simulink model "gm_uz_d_inverter_adapter"  (R2024b)
settings: Solver=FixedStepDiscrete  StartTime=0.0  StopTime=300e-5  RelTol=1e-3
undefined symbols (not defined in the file or in its folder): t_clk, t_clk_sig
libraries: hdlsllib x16, simulink x12
settings Model: Creator=Michael Hoerner  LastModifiedBy=hufnagelde
settings SolverCC: AlgebraicLoopSolver=TrustRegion
settings DataIOCC: LimitDataPoints=on  SaveOutput=off  SaveTime=off
settings OptimizationCC: BlockReduction=off  ConditionallyExecuteInputs=off  DefaultParameterBehavior=Inlined  LifeSpan=inf
settings DebuggingCC: AlgebraicLoopMsg=error  InheritedTsInSrcMsg=none  SingleTaskRateTransMsg=warning  UnconnectedInputMsg=warning  UnconnectedOutputMsg=warning  UnconnectedLineMsg=warning  AllowSymbolicDim=off  StrictBusMsg=ErrorOnBusTreatedAsVector  SFUnexpectedBacktrackingDiag=warning  SFNoUnconditionalDefaultTransitionDiag=warning  SFExecutionAtInitializationDiag=none  ArithmeticOperatorsInVariantConditions=warning
settings HardwareCC: ProdBitPerPointer=32  ProdBitPerSizeT=32  ProdBitPerPtrDiffT=32  ProdLargestAtomicFloat=None  ProdIntDivRoundTo=Undefined  ProdEndianess=Unspecified  ProdWordSize=32  ProdHWDeviceType=ASIC/FPGA->ASIC/FPGA  ProdEqTarget=off
settings ModelReferenceCC: EnableRefExpFcnMdlSchedulingChecks=on
settings SFSimCC: SimUseLocalCustomCode=off  CustomCodeUndefinedFunction=UseInterfaceOnly
settings RTWCC: RTWUseLocalCustomCode=off  GPUComputeCapability=3.5  DLArmComputeVersion=19.05
settings CodeAppCC: StateflowObjectComments=on
settings GRTTargetCC: TargetLangStandard=C89/C90 (ANSI)
settings ConfigComp: CovScope=ReferencedModels  CovMetricSettings=dw  CovSaveCumulativeToWorkspaceVar=on  CovSaveSingleToWorkspaceVar=on  CovExternalEMLEnable=off  CovSFcnEnable=off

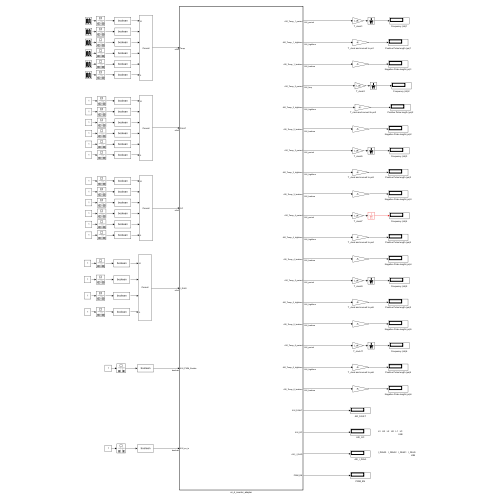
[thumbnail: Simulink's stored preview of the top-level diagram]
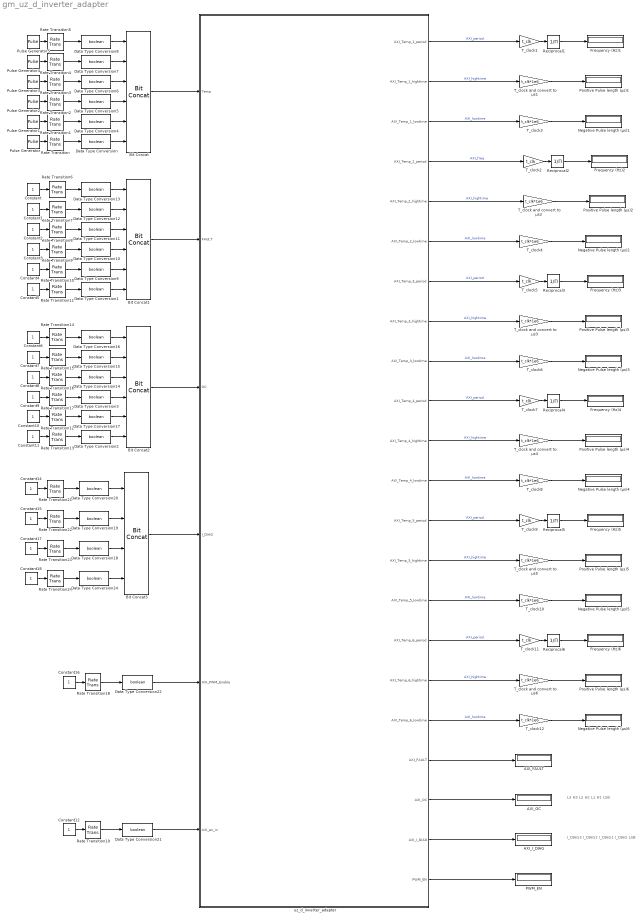
== system gm_uz_d_inverter_adapter ==
  note: I_DIAG3   I_DIAG2   I_DIAG1   I_DIAG
      |                                                        LSB
  note: L3   H3   L2   H2   L1   H1
      |                                   LSB
  AXI_FAULT : Display
      settings: Format=binary (Stored Integer)
  AXI_I_DIAG : Display
      settings: Format=binary (Stored Integer)
  AXI_OC : Display
      settings: Format=binary (Stored Integer)
  Bit Concat : hdlsllib/Logic and Bit Operations/Bit Concat  numInputs=6
  Bit Concat1 : hdlsllib/Logic and Bit Operations/Bit Concat  numInputs=6
  Bit Concat2 : hdlsllib/Logic and Bit Operations/Bit Concat  numInputs=6
  Bit Concat3 : hdlsllib/Logic and Bit Operations/Bit Concat  numInputs=4
  Constant{,1..12,14..18} (18 alike) : Constant
  Data Type Conversion{,1..22,24} (24 alike) : DataTypeConversion  OutDataTypeStr=boolean  SaturateOnIntegerOverflow=off  RndMeth=Floor
  Frequency (Hz){1..6} (6 alike) : Display
  Negative Pulse length (µs){1..6} (6 alike) : Display
  PWM_EN : Display
      settings: Format=decimal (Stored Integer)
  Positive Pulse length (µs){1..6} (6 alike) : Display
  Pulse Generator : DiscretePulseGenerator  PulseType=Time based  Period=t_clk_sig  PulseWidth=10
  Pulse Generator1 : DiscretePulseGenerator  PulseType=Time based  Period=t_clk_sig  PulseWidth=20
  Pulse Generator2 : DiscretePulseGenerator  PulseType=Time based  Period=t_clk_sig  PulseWidth=30
  Pulse Generator3 : DiscretePulseGenerator  PulseType=Time based  Period=t_clk_sig  PulseWidth=40
  Pulse Generator4 : DiscretePulseGenerator  PulseType=Time based  Period=t_clk_sig  PulseWidth=50
  Pulse Generator5 : DiscretePulseGenerator  PulseType=Time based  Period=t_clk_sig  PulseWidth=60
  Rate Transition{,1..5} (6 alike) : RateTransition  Deterministic=off  OutPortSampleTime=t_clk
  Rate Transition{6..19,21..24} (18 alike) : RateTransition  OutPortSampleTime=t_clk
  Reciprocal{1..6} (6 alike) : Product  Inputs=/
  T_clock and convert to µs{1..6} (6 alike) : Gain  Gain=t_clk*1e6
  T_clock{1..2,5,7,9,11} (6 alike) : Gain  Gain=t_clk
  T_clock{3..4,6,8,10,12} (6 alike) : Gain  Gain=t_clk*1e6
  uz_d_inverter_adapter : Subsystem  TreatAsAtomicUnit=on
  wires:
  Data Type Conversion21/1 -> uz_d_inverter_adapter/6(AXI_en_in)
  Rate Transition19/1 -> Data Type Conversion21/1
  Constant12/1 -> Rate Transition19/1
  uz_d_inverter_adapter/22(PWM_EN) -> PWM_EN/1
  uz_d_inverter_adapter/21(AXI_I_DIAG) -> AXI_I_DIAG/1
  uz_d_inverter_adapter/20(AXI_OC) -> AXI_OC/1
  Bit Concat3/1 -> uz_d_inverter_adapter/4(I_DIAG)
  Data Type Conversion24/1 -> Bit Concat3/4
  Data Type Conversion18/1 -> Bit Concat3/3
  Data Type Conversion19/1 -> Bit Concat3/2
  Data Type Conversion20/1 -> Bit Concat3/1
  Rate Transition23/1 -> Data Type Conversion18/1
  Rate Transition21/1 -> Data Type Conversion20/1
  Rate Transition24/1 -> Data Type Conversion24/1
  Constant17/1 -> Rate Transition23/1
  Constant14/1 -> Rate Transition21/1
  Rate Transition22/1 -> Data Type Conversion19/1
  Constant15/1 -> Rate Transition22/1
  Constant18/1 -> Rate Transition24/1
  Bit Concat2/1 -> uz_d_inverter_adapter/3(OC)
  Data Type Conversion2/1 -> Bit Concat2/6
  Constant7/1 -> Rate Transition15/1
  Rate Transition15/1 -> Data Type Conversion15/1
  Constant9/1 -> Rate Transition17/1
  Data Type Conversion17/1 -> Bit Concat2/5
  Constant10/1 -> Rate Transition12/1
  Constant11/1 -> Rate Transition13/1
  Constant8/1 -> Rate Transition16/1
  Constant6/1 -> Rate Transition14/1
  Rate Transition12/1 -> Data Type Conversion17/1
  Data Type Conversion15/1 -> Bit Concat2/2
  Data Type Conversion14/1 -> Bit Concat2/3
  Data Type Conversion3/1 -> Bit Concat2/4
  Rate Transition13/1 -> Data Type Conversion2/1
  Rate Transition14/1 -> Data Type Conversion16/1
  Rate Transition17/1 -> Data Type Conversion3/1
  Rate Transition16/1 -> Data Type Conversion14/1
  Data Type Conversion16/1 -> Bit Concat2/1
  Data Type Conversion22/1 -> uz_d_inverter_adapter/5(AXI_PWM_Enable)
  Rate Transition11/1 -> Data Type Conversion1/1
  Rate Transition10/1 -> Data Type Conversion9/1
  Rate Transition9/1 -> Data Type Conversion10/1
  Rate Transition8/1 -> Data Type Conversion11/1
  Rate Transition7/1 -> Data Type Conversion12/1
  Rate Transition6/1 -> Data Type Conversion13/1
  Bit Concat1/1 -> uz_d_inverter_adapter/2(FAULT)
  Data Type Conversion1/1 -> Bit Concat1/6
  Data Type Conversion13/1 -> Bit Concat1/1
  Data Type Conversion12/1 -> Bit Concat1/2
  Data Type Conversion9/1 -> Bit Concat1/5
  Data Type Conversion10/1 -> Bit Concat1/4
  Data Type Conversion11/1 -> Bit Concat1/3
  Data Type Conversion4/1 -> Bit Concat/5
  Data Type Conversion/1 -> Bit Concat/6
  Rate Transition5/1 -> Data Type Conversion8/1
  Rate Transition4/1 -> Data Type Conversion7/1
  Rate Transition3/1 -> Data Type Conversion6/1
  Rate Transition2/1 -> Data Type Conversion5/1
  Rate Transition1/1 -> Data Type Conversion4/1
  Bit Concat/1 -> uz_d_inverter_adapter/1(Temp)
  Rate Transition18/1 -> Data Type Conversion22/1
  Constant16/1 -> Rate Transition18/1
  Data Type Conversion8/1 -> Bit Concat/1
  Data Type Conversion7/1 -> Bit Concat/2
  Data Type Conversion6/1 -> Bit Concat/3
  Data Type Conversion5/1 -> Bit Concat/4
  uz_d_inverter_adapter/19(AXI_FAULT) -> AXI_FAULT/1
  uz_d_inverter_adapter/16(AXI_Temp_6_period) -> T_clock11/1  "AXI_period"
  T_clock and convert to µs6/1 -> Positive Pulse length (µs)6/1
  uz_d_inverter_adapter/17(AXI_Temp_6_hightime) -> T_clock and convert to µs6/1  "AXI_hightime"
  T_clock12/1 -> Negative Pulse length (µs)6/1
  Reciprocal6/1 -> Frequency (Hz)6/1
  T_clock11/1 -> Reciprocal6/1
  uz_d_inverter_adapter/18(AXI_Temp_6_lowtime) -> T_clock12/1  "AXI_lowtime"
  uz_d_inverter_adapter/13(AXI_Temp_5_period) -> T_clock9/1  "AXI_period"
  T_clock and convert to µs5/1 -> Positive Pulse length (µs)5/1
  uz_d_inverter_adapter/14(AXI_Temp_5_hightime) -> T_clock and convert to µs5/1  "AXI_hightime"
  T_clock10/1 -> Negative Pulse length (µs)5/1
  Reciprocal5/1 -> Frequency (Hz)5/1
  T_clock9/1 -> Reciprocal5/1
  uz_d_inverter_adapter/15(AXI_Temp_5_lowtime) -> T_clock10/1  "AXI_lowtime"
  uz_d_inverter_adapter/10(AXI_Temp_4_period) -> T_clock7/1  "AXI_period"
  T_clock and convert to µs4/1 -> Positive Pulse length (µs)4/1
  uz_d_inverter_adapter/11(AXI_Temp_4_hightime) -> T_clock and convert to µs4/1  "AXI_hightime"
  T_clock8/1 -> Negative Pulse length (µs)4/1
  Reciprocal4/1 -> Frequency (Hz)4/1
  T_clock7/1 -> Reciprocal4/1
  uz_d_inverter_adapter/12(AXI_Temp_4_lowtime) -> T_clock8/1  "AXI_lowtime"
  uz_d_inverter_adapter/7(AXI_Temp_3_period) -> T_clock5/1  "AXI_period"
  T_clock and convert to µs3/1 -> Positive Pulse length (µs)3/1
  uz_d_inverter_adapter/8(AXI_Temp_3_hightime) -> T_clock and convert to µs3/1  "AXI_hightime"
  T_clock6/1 -> Negative Pulse length (µs)3/1
  Reciprocal3/1 -> Frequency (Hz)3/1
  T_clock5/1 -> Reciprocal3/1
  uz_d_inverter_adapter/9(AXI_Temp_3_lowtime) -> T_clock6/1  "AXI_lowtime"
  uz_d_inverter_adapter/4(AXI_Temp_2_period) -> T_clock2/1  "AXI_freq"
  T_clock and convert to µs2/1 -> Positive Pulse length (µs)2/1
  uz_d_inverter_adapter/5(AXI_Temp_2_hightime) -> T_clock and convert to µs2/1  "AXI_hightime"
  T_clock4/1 -> Negative Pulse length (µs)2/1
  Reciprocal2/1 -> Frequency (Hz)2/1
  T_clock2/1 -> Reciprocal2/1
  uz_d_inverter_adapter/6(AXI_Temp_2_lowtime) -> T_clock4/1  "AXI_lowtime"
  uz_d_inverter_adapter/1(AXI_Temp_1_period) -> T_clock1/1  "AXI_period"
  T_clock1/1 -> Reciprocal1/1
  uz_d_inverter_adapter/2(AXI_Temp_1_hightime) -> T_clock and convert to µs1/1  "AXI_hightime"
  uz_d_inverter_adapter/3(AXI_Temp_1_lowtime) -> T_clock3/1  "AXI_lowtime"
  Reciprocal1/1 -> Frequency (Hz)1/1
  T_clock3/1 -> Negative Pulse length (µs)1/1
  T_clock and convert to µs1/1 -> Positive Pulse length (µs)1/1
  Constant5/1 -> Rate Transition11/1
  Constant4/1 -> Rate Transition10/1
  Constant3/1 -> Rate Transition9/1
  Constant2/1 -> Rate Transition8/1
  Constant1/1 -> Rate Transition7/1
  Constant/1 -> Rate Transition6/1
  Rate Transition/1 -> Data Type Conversion/1
  Pulse Generator5/1 -> Rate Transition5/1
  Pulse Generator4/1 -> Rate Transition4/1
  Pulse Generator3/1 -> Rate Transition3/1
  Pulse Generator2/1 -> Rate Transition2/1
  Pulse Generator1/1 -> Rate Transition1/1
  Pulse Generator/1 -> Rate Transition/1

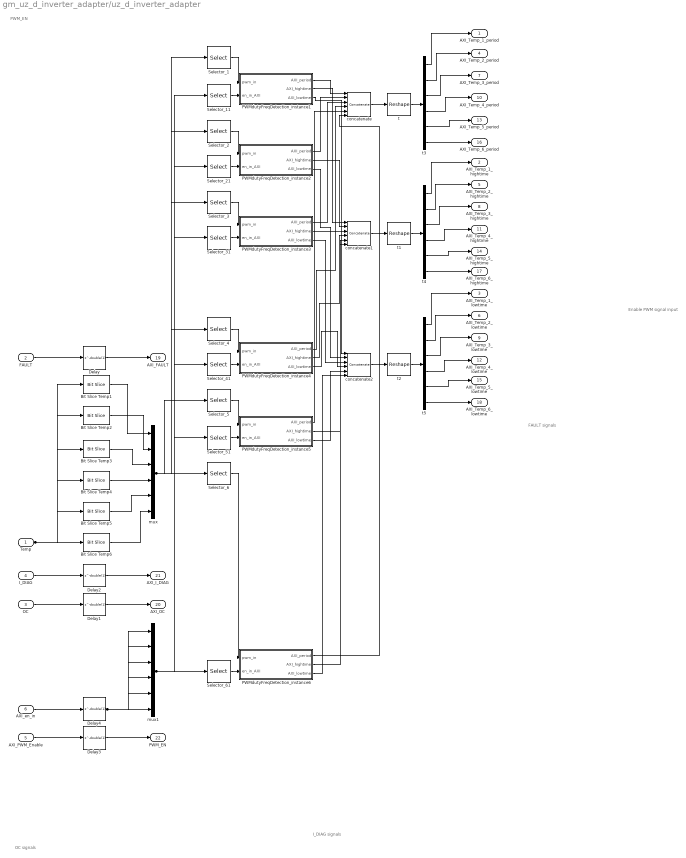
== system gm_uz_d_inverter_adapter/uz_d_inverter_adapter ==
  note: PWM_EN
  note: I_DIAG signals
  note: FAULT signals
  note: OC signals
  note: Enable PWM signal input
  Temp : Inport  OutDataTypeStr=fixdt(0, 6, 0)  PortDimensions=1  SampleTime=1e-08
  FAULT : Inport  Port=2  OutDataTypeStr=fixdt(0, 6, 0)  PortDimensions=1  SampleTime=1e-08
  OC : Inport  Port=3  OutDataTypeStr=fixdt(0, 6, 0)  PortDimensions=1  SampleTime=1e-08
  I_DIAG : Inport  Port=4  OutDataTypeStr=fixdt(0, 4, 0)  PortDimensions=1  SampleTime=1e-08
  AXI_PWM_Enable : Inport  Port=5  OutDataTypeStr=boolean  PortDimensions=1  SampleTime=1e-08
  AXI_en_in : Inport  Port=6  OutDataTypeStr=boolean  PortDimensions=1  SampleTime=1e-08
  Bit Slice Temp1 : hdlsllib/Logic and Bit Operations/Bit Slice  lidx=double(0)  ridx=double(0)
  Bit Slice Temp2 : hdlsllib/Logic and Bit Operations/Bit Slice  lidx=double(1)  ridx=double(1)
  Bit Slice Temp3 : hdlsllib/Logic and Bit Operations/Bit Slice  lidx=double(2)  ridx=double(2)
  Bit Slice Temp4 : hdlsllib/Logic and Bit Operations/Bit Slice  lidx=double(3)  ridx=double(3)
  Bit Slice Temp5 : hdlsllib/Logic and Bit Operations/Bit Slice  lidx=double(4)  ridx=double(4)
  Bit Slice Temp6 : hdlsllib/Logic and Bit Operations/Bit Slice  lidx=double(5)  ridx=double(5)
  Delay{,1..4} (5 alike) : Delay  DelayLength=double(1)  InitialCondition=0  SampleTime=1e-08
  PWMdutyFreqDetection_instance1 : Subsystem
  PWMdutyFreqDetection_instance2 : Subsystem
  PWMdutyFreqDetection_instance3 : Subsystem
  PWMdutyFreqDetection_instance4 : Subsystem
  PWMdutyFreqDetection_instance5 : Subsystem
  PWMdutyFreqDetection_instance6 : Subsystem
  Selector_1 : Selector  InputPortWidth=6  IndexOptions=Index vector (dialog)  Indices=double(1)  OutputSizes=1
  Selector_11 : Selector  InputPortWidth=6  IndexOptions=Index vector (dialog)  Indices=double(1)  OutputSizes=1
  Selector_2 : Selector  InputPortWidth=6  IndexOptions=Index vector (dialog)  Indices=double(2)  OutputSizes=1
  Selector_21 : Selector  InputPortWidth=6  IndexOptions=Index vector (dialog)  Indices=double(2)  OutputSizes=1
  Selector_3 : Selector  InputPortWidth=6  IndexOptions=Index vector (dialog)  Indices=double(3)  OutputSizes=1
  Selector_31 : Selector  InputPortWidth=6  IndexOptions=Index vector (dialog)  Indices=double(3)  OutputSizes=1
  Selector_4 : Selector  InputPortWidth=6  IndexOptions=Index vector (dialog)  Indices=double(4)  OutputSizes=1
  Selector_41 : Selector  InputPortWidth=6  IndexOptions=Index vector (dialog)  Indices=double(4)  OutputSizes=1
  Selector_5 : Selector  InputPortWidth=6  IndexOptions=Index vector (dialog)  Indices=double(5)  OutputSizes=1
  Selector_51 : Selector  InputPortWidth=6  IndexOptions=Index vector (dialog)  Indices=double(5)  OutputSizes=1
  Selector_6 : Selector  InputPortWidth=6  IndexOptions=Index vector (dialog)  Indices=double(6)  OutputSizes=1
  Selector_61 : Selector  InputPortWidth=6  IndexOptions=Index vector (dialog)  Indices=double(6)  OutputSizes=1
  concatenate : Concatenate  NumInputs=6
  concatenate1 : Concatenate  NumInputs=6
  concatenate2 : Concatenate  NumInputs=6
  mux : Mux  Inputs=6
  mux1 : Mux  Inputs=6
  t : Reshape
  t1 : Reshape
  t2 : Reshape
  t3 : Demux  Outputs=6
  t4 : Demux  Outputs=6
  t5 : Demux  Outputs=6
  AXI_Temp_1_period : Outport  PortDimensions=1  SampleTime=1e-08  VectorParamsAs1DForOutWhenUnconnected=off
  AXI_Temp_1_hightime : Outport  Port=2  PortDimensions=1  SampleTime=1e-08  VectorParamsAs1DForOutWhenUnconnected=off
  AXI_Temp_1_lowtime : Outport  Port=3  PortDimensions=1  SampleTime=1e-08  VectorParamsAs1DForOutWhenUnconnected=off
  AXI_Temp_2_period : Outport  Port=4  PortDimensions=1  SampleTime=1e-08  VectorParamsAs1DForOutWhenUnconnected=off
  AXI_Temp_2_hightime : Outport  Port=5  PortDimensions=1  SampleTime=1e-08  VectorParamsAs1DForOutWhenUnconnected=off
  AXI_Temp_2_lowtime : Outport  Port=6  PortDimensions=1  SampleTime=1e-08  VectorParamsAs1DForOutWhenUnconnected=off
  AXI_Temp_3_period : Outport  Port=7  PortDimensions=1  SampleTime=1e-08  VectorParamsAs1DForOutWhenUnconnected=off
  AXI_Temp_3_hightime : Outport  Port=8  PortDimensions=1  SampleTime=1e-08  VectorParamsAs1DForOutWhenUnconnected=off
  AXI_Temp_3_lowtime : Outport  Port=9  PortDimensions=1  SampleTime=1e-08  VectorParamsAs1DForOutWhenUnconnected=off
  AXI_Temp_4_period : Outport  Port=10  PortDimensions=1  SampleTime=1e-08  VectorParamsAs1DForOutWhenUnconnected=off
  AXI_Temp_4_hightime : Outport  Port=11  PortDimensions=1  SampleTime=1e-08  VectorParamsAs1DForOutWhenUnconnected=off
  AXI_Temp_4_lowtime : Outport  Port=12  PortDimensions=1  SampleTime=1e-08  VectorParamsAs1DForOutWhenUnconnected=off
  AXI_Temp_5_period : Outport  Port=13  PortDimensions=1  SampleTime=1e-08  VectorParamsAs1DForOutWhenUnconnected=off
  AXI_Temp_5_hightime : Outport  Port=14  PortDimensions=1  SampleTime=1e-08  VectorParamsAs1DForOutWhenUnconnected=off
  AXI_Temp_5_lowtime : Outport  Port=15  PortDimensions=1  SampleTime=1e-08  VectorParamsAs1DForOutWhenUnconnected=off
  AXI_Temp_6_period : Outport  Port=16  PortDimensions=1  SampleTime=1e-08  VectorParamsAs1DForOutWhenUnconnected=off
  AXI_Temp_6_hightime : Outport  Port=17  PortDimensions=1  SampleTime=1e-08  VectorParamsAs1DForOutWhenUnconnected=off
  AXI_Temp_6_lowtime : Outport  Port=18  PortDimensions=1  SampleTime=1e-08  VectorParamsAs1DForOutWhenUnconnected=off
  AXI_FAULT : Outport  Port=19  PortDimensions=1  SampleTime=1e-08  VectorParamsAs1DForOutWhenUnconnected=off
  AXI_OC : Outport  Port=20  PortDimensions=1  SampleTime=1e-08  VectorParamsAs1DForOutWhenUnconnected=off
  AXI_I_DIAG : Outport  Port=21  PortDimensions=1  SampleTime=1e-08  VectorParamsAs1DForOutWhenUnconnected=off
  PWM_EN : Outport  Port=22  PortDimensions=1  SampleTime=1e-08  VectorParamsAs1DForOutWhenUnconnected=off
  wires:
  PWMdutyFreqDetection_instance4/3(AXI_lowtime) -> concatenate2/4
  Delay/1 -> AXI_FAULT/1
  t3/2 -> AXI_Temp_2_period/1
  PWMdutyFreqDetection_instance3/1(AXI_period) -> concatenate/3
  t3/1 -> AXI_Temp_1_period/1
  FAULT/1 -> Delay/1
  PWMdutyFreqDetection_instance4/1(AXI_period) -> concatenate/4
  Selector_51/1 -> PWMdutyFreqDetection_instance5/2(en_in_AXI)
  Temp/1 -> Bit Slice Temp6/1, Bit Slice Temp5/1, Bit Slice Temp4/1, Bit Slice Temp3/1, Bit Slice Temp1/1, Bit Slice Temp2/1
  AXI_en_in/1 -> Delay4/1
  I_DIAG/1 -> Delay2/1
  OC/1 -> Delay1/1
  AXI_PWM_Enable/1 -> Delay3/1
  Selector_21/1 -> PWMdutyFreqDetection_instance2/2(en_in_AXI)
  Bit Slice Temp1/1 -> mux/1
  Bit Slice Temp2/1 -> mux/2
  Bit Slice Temp3/1 -> mux/3
  Selector_11/1 -> PWMdutyFreqDetection_instance1/2(en_in_AXI)
  Bit Slice Temp4/1 -> mux/4
  PWMdutyFreqDetection_instance2/1(AXI_period) -> concatenate/2
  Bit Slice Temp5/1 -> mux/5
  PWMdutyFreqDetection_instance6/2(AXI_hightime) -> concatenate1/6
  Bit Slice Temp6/1 -> mux/6
  Selector_4/1 -> PWMdutyFreqDetection_instance4/1(pwm_in)
  Delay2/1 -> AXI_I_DIAG/1
  t3/4 -> AXI_Temp_4_period/1
  Delay1/1 -> AXI_OC/1
  t3/3 -> AXI_Temp_3_period/1
  Selector_6/1 -> PWMdutyFreqDetection_instance6/1(pwm_in)
  Delay4/1 -> mux1/3, mux1/2, mux1/1, mux1/4, mux1/5, mux1/6
  Delay3/1 -> PWM_EN/1
  mux/1 -> Selector_3/1, Selector_6/1, Selector_2/1, Selector_1/1, Selector_4/1, Selector_5/1
  mux1/1 -> Selector_61/1, Selector_41/1, Selector_51/1, Selector_21/1, Selector_11/1, Selector_31/1
  Selector_1/1 -> PWMdutyFreqDetection_instance1/1(pwm_in)
  PWMdutyFreqDetection_instance5/2(AXI_hightime) -> concatenate1/5
  Selector_2/1 -> PWMdutyFreqDetection_instance2/1(pwm_in)
  Selector_3/1 -> PWMdutyFreqDetection_instance3/1(pwm_in)
  Selector_31/1 -> PWMdutyFreqDetection_instance3/2(en_in_AXI)
  Selector_41/1 -> PWMdutyFreqDetection_instance4/2(en_in_AXI)
  Selector_5/1 -> PWMdutyFreqDetection_instance5/1(pwm_in)
  t3/6 -> AXI_Temp_6_period/1
  t3/5 -> AXI_Temp_5_period/1
  Selector_61/1 -> PWMdutyFreqDetection_instance6/2(en_in_AXI)
  PWMdutyFreqDetection_instance1/1(AXI_period) -> concatenate/1
  PWMdutyFreqDetection_instance1/2(AXI_hightime) -> concatenate1/1
  PWMdutyFreqDetection_instance5/3(AXI_lowtime) -> concatenate2/5
  PWMdutyFreqDetection_instance1/3(AXI_lowtime) -> concatenate2/1
  PWMdutyFreqDetection_instance6/1(AXI_period) -> concatenate/6
  PWMdutyFreqDetection_instance2/2(AXI_hightime) -> concatenate1/2
  PWMdutyFreqDetection_instance6/3(AXI_lowtime) -> concatenate2/6
  PWMdutyFreqDetection_instance2/3(AXI_lowtime) -> concatenate2/2
  PWMdutyFreqDetection_instance3/2(AXI_hightime) -> concatenate1/3
  PWMdutyFreqDetection_instance3/3(AXI_lowtime) -> concatenate2/3
  PWMdutyFreqDetection_instance4/2(AXI_hightime) -> concatenate1/4
  PWMdutyFreqDetection_instance5/1(AXI_period) -> concatenate/5
  concatenate/1 -> t/1
  concatenate1/1 -> t1/1
  concatenate2/1 -> t2/1
  t/1 -> t3/1
  t1/1 -> t4/1
  t2/1 -> t5/1
  t4/2 -> AXI_Temp_2_hightime/1
  t4/1 -> AXI_Temp_1_hightime/1
  t4/3 -> AXI_Temp_3_hightime/1
  t4/4 -> AXI_Temp_4_hightime/1
  t4/5 -> AXI_Temp_5_hightime/1
  t4/6 -> AXI_Temp_6_hightime/1
  t5/1 -> AXI_Temp_1_lowtime/1
  t5/2 -> AXI_Temp_2_lowtime/1
  t5/3 -> AXI_Temp_3_lowtime/1
  t5/4 -> AXI_Temp_4_lowtime/1
  t5/5 -> AXI_Temp_5_lowtime/1
  t5/6 -> AXI_Temp_6_lowtime/1

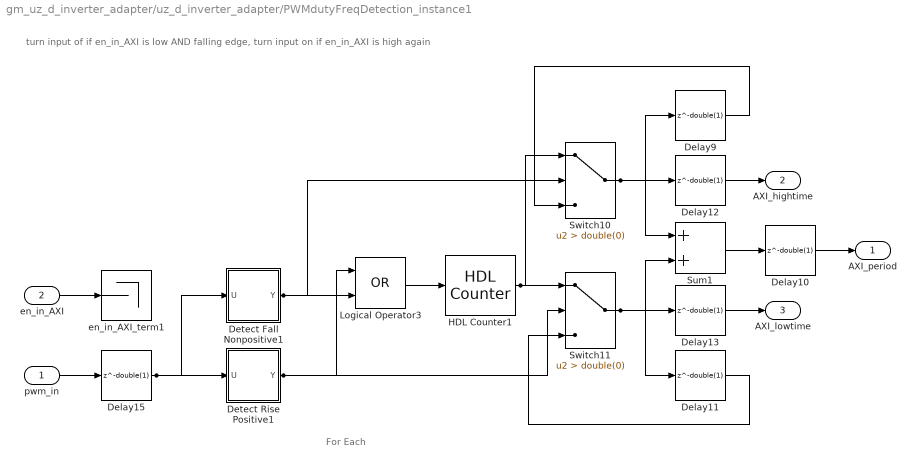
== system gm_uz_d_inverter_adapter/uz_d_inverter_adapter/PWMdutyFreqDetection_instance1 ==
  note: For Each
  note: turn input of if en_in_AXI is low AND falling edge, turn input on if en_in_AXI is high again
  pwm_in : Inport  OutDataTypeStr=fixdt(0, 1, 0)  PortDimensions=1  SampleTime=1e-08
  en_in_AXI : Inport  Port=2  OutDataTypeStr=boolean  PortDimensions=1  SampleTime=1e-08
  Delay{9..13,15} (6 alike) : Delay  DelayLength=double(1)  InitialCondition=0  SampleTime=1e-08
  Detect Fall Nonpositive1 : Subsystem  mask(Detect Fall Nonpositive){vinit=double(0), InputProcessing=Elements as channels (sample based), OutDataTypeStr=boolean}
      mask prompts: vinit "Simulink:masks:InitialCondition_MP"; InputProcessing "Simulink:masks:InputProcessing_MP"; OutDataTypeStr "Simulink:masks:OutputDataType_MP"
      mask help: Simulink:masks:DetectFallNonpositive_MD
      mask init:
      | InputProcessing = 'Elements as channels (sample based)';
      | OutDataTypeStr = 'boolean';
      | vinit = double(0);
      mask TypeOptions InputProcessing: Simulink:masks:ColumnsAsChannelsFrameBased | Simulink:masks:ElementsAsChannelsSampleBased
      mask TypeOptions OutDataTypeStr: Simulink:masks:uint8 | Simulink:masks:boolean
      mask Display: fprintf('U <= 0\n&  NOT\nU/z <= 0')
  Detect Rise Positive1 : Subsystem  mask(Detect Rise Positive){vinit=double(0), InputProcessing=Elements as channels (sample based), OutDataTypeStr=boolean}
      mask prompts: vinit "Simulink:masks:InitialCondition_MP"; InputProcessing "Simulink:masks:InputProcessing_MP"; OutDataTypeStr "Simulink:masks:OutputDataType_MP"
      mask help: Simulink:masks:DetectRisePositive_MD
      mask init:
      | InputProcessing = 'Elements as channels (sample based)';
      | OutDataTypeStr = 'boolean';
      | vinit = double(0);
      mask TypeOptions InputProcessing: Simulink:masks:ColumnsAsChannelsFrameBased | Simulink:masks:ElementsAsChannelsSampleBased
      mask TypeOptions OutDataTypeStr: Simulink:masks:uint8 | Simulink:masks:boolean
      mask Display: fprintf('U > 0\n&  NOT\nU/z > 0')
  HDL Counter1 : hdlsllib/Sources/HDL Counter  CountType=Count limited  CountInit=1  CountStep=1  CountMax=2500000  CountFromType=Specify  CountFrom=1  CountResetPort=on  CountLoadPort=off  CountEnbPort=off  CountDirPort=off  CountHitOutputPort=off  CountDataType=Unsigned  CountWordLen=32  CountFracLen=0  CountSampTime=1
  Logical Operator3 : Logic  Operator=OR  AllPortsSameDT=off  OutDataTypeStr=boolean  SampleTime=1e-08
  Sum1 : Sum  OutDataTypeStr=uint32  AccumDataTypeStr=uint32  SampleTime=1e-08
  Switch10 : Switch  Criteria=u2 > Threshold  Threshold=double(0)  OutDataTypeStr=uint32  SampleTime=1e-08  SaturateOnIntegerOverflow=off  InputSameDT=off
  Switch11 : Switch  Criteria=u2 > Threshold  Threshold=double(0)  OutDataTypeStr=uint32  SampleTime=1e-08  SaturateOnIntegerOverflow=off  InputSameDT=off
  en_in_AXI_term1 : Terminator
  AXI_period : Outport  SampleTime=1e-08
  AXI_hightime : Outport  Port=2  SampleTime=1e-08
  AXI_lowtime : Outport  Port=3  SampleTime=1e-08
  wires:
  en_in_AXI/1 -> en_in_AXI_term1/1
  Detect Fall Nonpositive1/1(Y) -> Switch10/2, Logical Operator3/2
  pwm_in/1 -> Delay15/1
  Switch10/1 -> Sum1/1, Delay12/1, Delay9/1
  Delay12/1 -> AXI_hightime/1
  Logical Operator3/1 -> HDL Counter1/1
  Delay15/1 -> Detect Fall Nonpositive1/1(U), Detect Rise Positive1/1(U)
  Detect Rise Positive1/1(Y) -> Switch11/2, Logical Operator3/1
  HDL Counter1/1 -> Switch10/1, Switch11/1
  Delay13/1 -> AXI_lowtime/1
  Switch11/1 -> Sum1/2, Delay13/1, Delay11/1
  Delay9/1 -> Switch10/3
  Sum1/1 -> Delay10/1
  Delay11/1 -> Switch11/3
  Delay10/1 -> AXI_period/1

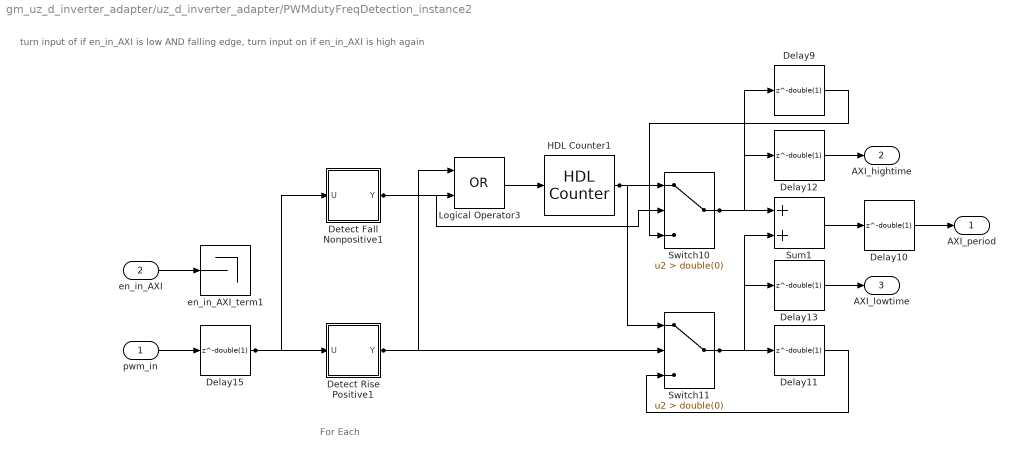
== system gm_uz_d_inverter_adapter/uz_d_inverter_adapter/PWMdutyFreqDetection_instance2 ==
  note: For Each
  note: turn input of if en_in_AXI is low AND falling edge, turn input on if en_in_AXI is high again
  pwm_in : Inport  OutDataTypeStr=fixdt(0, 1, 0)  PortDimensions=1  SampleTime=1e-08
  en_in_AXI : Inport  Port=2  OutDataTypeStr=boolean  PortDimensions=1  SampleTime=1e-08
  Delay{9..13,15} (6 alike) : Delay  DelayLength=double(1)  InitialCondition=0  SampleTime=1e-08
  Detect Fall Nonpositive1 : Subsystem  mask(Detect Fall Nonpositive){vinit=double(0), InputProcessing=Elements as channels (sample based), OutDataTypeStr=boolean}
      mask prompts: vinit "Simulink:masks:InitialCondition_MP"; InputProcessing "Simulink:masks:InputProcessing_MP"; OutDataTypeStr "Simulink:masks:OutputDataType_MP"
      mask help: Simulink:masks:DetectFallNonpositive_MD
      mask init:
      | InputProcessing = 'Elements as channels (sample based)';
      | OutDataTypeStr = 'boolean';
      | vinit = double(0);
      mask TypeOptions InputProcessing: Simulink:masks:ColumnsAsChannelsFrameBased | Simulink:masks:ElementsAsChannelsSampleBased
      mask TypeOptions OutDataTypeStr: Simulink:masks:uint8 | Simulink:masks:boolean
      mask Display: fprintf('U <= 0\n&  NOT\nU/z <= 0')
  Detect Rise Positive1 : Subsystem  mask(Detect Rise Positive){vinit=double(0), InputProcessing=Elements as channels (sample based), OutDataTypeStr=boolean}
      mask prompts: vinit "Simulink:masks:InitialCondition_MP"; InputProcessing "Simulink:masks:InputProcessing_MP"; OutDataTypeStr "Simulink:masks:OutputDataType_MP"
      mask help: Simulink:masks:DetectRisePositive_MD
      mask init:
      | InputProcessing = 'Elements as channels (sample based)';
      | OutDataTypeStr = 'boolean';
      | vinit = double(0);
      mask TypeOptions InputProcessing: Simulink:masks:ColumnsAsChannelsFrameBased | Simulink:masks:ElementsAsChannelsSampleBased
      mask TypeOptions OutDataTypeStr: Simulink:masks:uint8 | Simulink:masks:boolean
      mask Display: fprintf('U > 0\n&  NOT\nU/z > 0')
  HDL Counter1 : hdlsllib/Sources/HDL Counter  CountType=Count limited  CountInit=1  CountStep=1  CountMax=2500000  CountFromType=Specify  CountFrom=1  CountResetPort=on  CountLoadPort=off  CountEnbPort=off  CountDirPort=off  CountHitOutputPort=off  CountDataType=Unsigned  CountWordLen=32  CountFracLen=0  CountSampTime=1
  Logical Operator3 : Logic  Operator=OR  AllPortsSameDT=off  OutDataTypeStr=boolean  SampleTime=1e-08
  Sum1 : Sum  OutDataTypeStr=uint32  AccumDataTypeStr=uint32  SampleTime=1e-08
  Switch10 : Switch  Criteria=u2 > Threshold  Threshold=double(0)  OutDataTypeStr=uint32  SampleTime=1e-08  SaturateOnIntegerOverflow=off  InputSameDT=off
  Switch11 : Switch  Criteria=u2 > Threshold  Threshold=double(0)  OutDataTypeStr=uint32  SampleTime=1e-08  SaturateOnIntegerOverflow=off  InputSameDT=off
  en_in_AXI_term1 : Terminator
  AXI_period : Outport  SampleTime=1e-08
  AXI_hightime : Outport  Port=2  SampleTime=1e-08
  AXI_lowtime : Outport  Port=3  SampleTime=1e-08
  wires:
  Detect Fall Nonpositive1/1(Y) -> Switch10/2, Logical Operator3/2
  Delay15/1 -> Detect Fall Nonpositive1/1(U), Detect Rise Positive1/1(U)
  en_in_AXI/1 -> en_in_AXI_term1/1
  pwm_in/1 -> Delay15/1
  Detect Rise Positive1/1(Y) -> Switch11/2, Logical Operator3/1
  Delay10/1 -> AXI_period/1
  Switch10/1 -> Delay12/1, Delay9/1, Sum1/1
  Logical Operator3/1 -> HDL Counter1/1
  HDL Counter1/1 -> Switch10/1, Switch11/1
  Switch11/1 -> Sum1/2, Delay11/1, Delay13/1
  Delay9/1 -> Switch10/3
  Delay12/1 -> AXI_hightime/1
  Sum1/1 -> Delay10/1
  Delay13/1 -> AXI_lowtime/1
  Delay11/1 -> Switch11/3

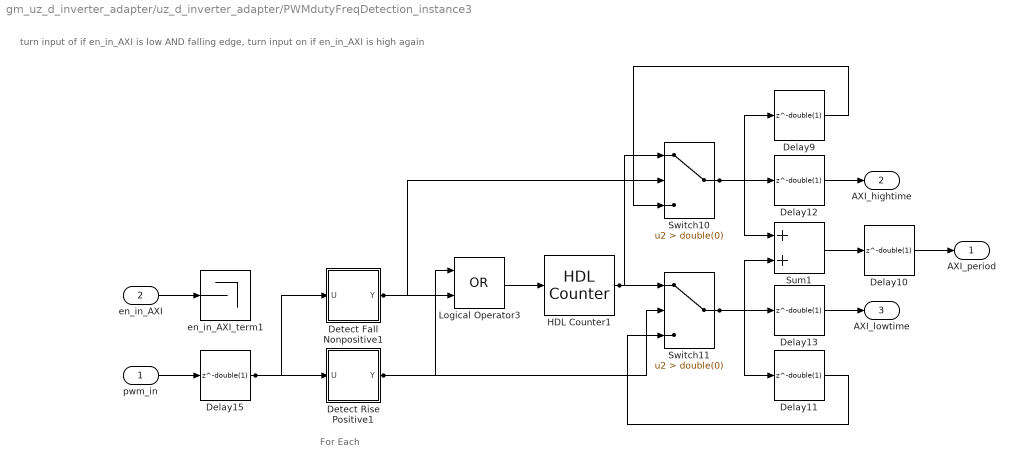
== system gm_uz_d_inverter_adapter/uz_d_inverter_adapter/PWMdutyFreqDetection_instance3 ==
  note: For Each
  note: turn input of if en_in_AXI is low AND falling edge, turn input on if en_in_AXI is high again
  pwm_in : Inport  OutDataTypeStr=fixdt(0, 1, 0)  PortDimensions=1  SampleTime=1e-08
  en_in_AXI : Inport  Port=2  OutDataTypeStr=boolean  PortDimensions=1  SampleTime=1e-08
  Delay{9..13,15} (6 alike) : Delay  DelayLength=double(1)  InitialCondition=0  SampleTime=1e-08
  Detect Fall Nonpositive1 : Subsystem  mask(Detect Fall Nonpositive){vinit=double(0), InputProcessing=Elements as channels (sample based), OutDataTypeStr=boolean}
      mask prompts: vinit "Simulink:masks:InitialCondition_MP"; InputProcessing "Simulink:masks:InputProcessing_MP"; OutDataTypeStr "Simulink:masks:OutputDataType_MP"
      mask help: Simulink:masks:DetectFallNonpositive_MD
      mask init:
      | InputProcessing = 'Elements as channels (sample based)';
      | OutDataTypeStr = 'boolean';
      | vinit = double(0);
      mask TypeOptions InputProcessing: Simulink:masks:ColumnsAsChannelsFrameBased | Simulink:masks:ElementsAsChannelsSampleBased
      mask TypeOptions OutDataTypeStr: Simulink:masks:uint8 | Simulink:masks:boolean
      mask Display: fprintf('U <= 0\n&  NOT\nU/z <= 0')
  Detect Rise Positive1 : Subsystem  mask(Detect Rise Positive){vinit=double(0), InputProcessing=Elements as channels (sample based), OutDataTypeStr=boolean}
      mask prompts: vinit "Simulink:masks:InitialCondition_MP"; InputProcessing "Simulink:masks:InputProcessing_MP"; OutDataTypeStr "Simulink:masks:OutputDataType_MP"
      mask help: Simulink:masks:DetectRisePositive_MD
      mask init:
      | InputProcessing = 'Elements as channels (sample based)';
      | OutDataTypeStr = 'boolean';
      | vinit = double(0);
      mask TypeOptions InputProcessing: Simulink:masks:ColumnsAsChannelsFrameBased | Simulink:masks:ElementsAsChannelsSampleBased
      mask TypeOptions OutDataTypeStr: Simulink:masks:uint8 | Simulink:masks:boolean
      mask Display: fprintf('U > 0\n&  NOT\nU/z > 0')
  HDL Counter1 : hdlsllib/Sources/HDL Counter  CountType=Count limited  CountInit=1  CountStep=1  CountMax=2500000  CountFromType=Specify  CountFrom=1  CountResetPort=on  CountLoadPort=off  CountEnbPort=off  CountDirPort=off  CountHitOutputPort=off  CountDataType=Unsigned  CountWordLen=32  CountFracLen=0  CountSampTime=1
  Logical Operator3 : Logic  Operator=OR  AllPortsSameDT=off  OutDataTypeStr=boolean  SampleTime=1e-08
  Sum1 : Sum  OutDataTypeStr=uint32  AccumDataTypeStr=uint32  SampleTime=1e-08
  Switch10 : Switch  Criteria=u2 > Threshold  Threshold=double(0)  OutDataTypeStr=uint32  SampleTime=1e-08  SaturateOnIntegerOverflow=off  InputSameDT=off
  Switch11 : Switch  Criteria=u2 > Threshold  Threshold=double(0)  OutDataTypeStr=uint32  SampleTime=1e-08  SaturateOnIntegerOverflow=off  InputSameDT=off
  en_in_AXI_term1 : Terminator
  AXI_period : Outport  SampleTime=1e-08
  AXI_hightime : Outport  Port=2  SampleTime=1e-08
  AXI_lowtime : Outport  Port=3  SampleTime=1e-08
  wires:
  en_in_AXI/1 -> en_in_AXI_term1/1
  pwm_in/1 -> Delay15/1
  Detect Fall Nonpositive1/1(Y) -> Switch10/2, Logical Operator3/2
  Delay15/1 -> Detect Fall Nonpositive1/1(U), Detect Rise Positive1/1(U)
  Detect Rise Positive1/1(Y) -> Switch11/2, Logical Operator3/1
  Switch10/1 -> Sum1/1, Delay12/1, Delay9/1
  Logical Operator3/1 -> HDL Counter1/1
  HDL Counter1/1 -> Switch10/1, Switch11/1
  Switch11/1 -> Sum1/2, Delay13/1, Delay11/1
  Delay9/1 -> Switch10/3
  Delay12/1 -> AXI_hightime/1
  Sum1/1 -> Delay10/1
  Delay13/1 -> AXI_lowtime/1
  Delay11/1 -> Switch11/3
  Delay10/1 -> AXI_period/1

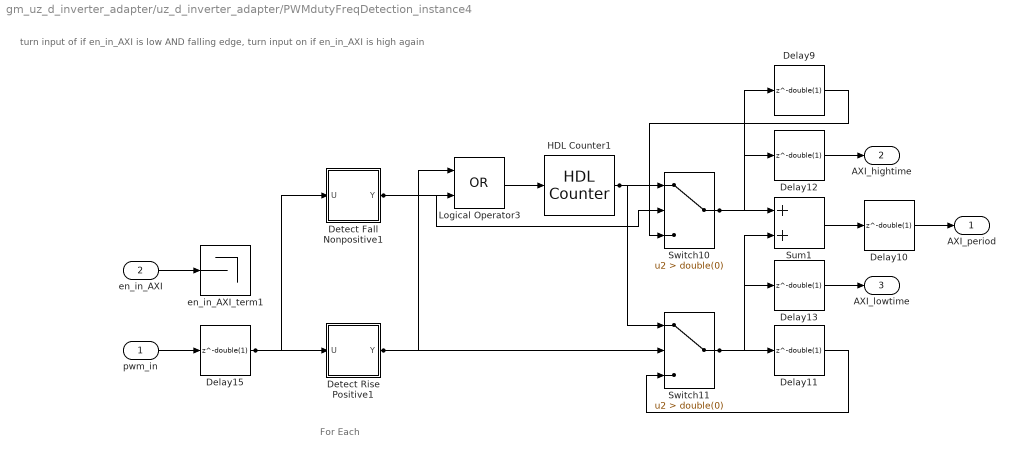
== system gm_uz_d_inverter_adapter/uz_d_inverter_adapter/PWMdutyFreqDetection_instance4 ==
  note: For Each
  note: turn input of if en_in_AXI is low AND falling edge, turn input on if en_in_AXI is high again
  pwm_in : Inport  OutDataTypeStr=fixdt(0, 1, 0)  PortDimensions=1  SampleTime=1e-08
  en_in_AXI : Inport  Port=2  OutDataTypeStr=boolean  PortDimensions=1  SampleTime=1e-08
  Delay{9..13,15} (6 alike) : Delay  DelayLength=double(1)  InitialCondition=0  SampleTime=1e-08
  Detect Fall Nonpositive1 : Subsystem  mask(Detect Fall Nonpositive){vinit=double(0), InputProcessing=Elements as channels (sample based), OutDataTypeStr=boolean}
      mask prompts: vinit "Simulink:masks:InitialCondition_MP"; InputProcessing "Simulink:masks:InputProcessing_MP"; OutDataTypeStr "Simulink:masks:OutputDataType_MP"
      mask help: Simulink:masks:DetectFallNonpositive_MD
      mask init:
      | InputProcessing = 'Elements as channels (sample based)';
      | OutDataTypeStr = 'boolean';
      | vinit = double(0);
      mask TypeOptions InputProcessing: Simulink:masks:ColumnsAsChannelsFrameBased | Simulink:masks:ElementsAsChannelsSampleBased
      mask TypeOptions OutDataTypeStr: Simulink:masks:uint8 | Simulink:masks:boolean
      mask Display: fprintf('U <= 0\n&  NOT\nU/z <= 0')
  Detect Rise Positive1 : Subsystem  mask(Detect Rise Positive){vinit=double(0), InputProcessing=Elements as channels (sample based), OutDataTypeStr=boolean}
      mask prompts: vinit "Simulink:masks:InitialCondition_MP"; InputProcessing "Simulink:masks:InputProcessing_MP"; OutDataTypeStr "Simulink:masks:OutputDataType_MP"
      mask help: Simulink:masks:DetectRisePositive_MD
      mask init:
      | InputProcessing = 'Elements as channels (sample based)';
      | OutDataTypeStr = 'boolean';
      | vinit = double(0);
      mask TypeOptions InputProcessing: Simulink:masks:ColumnsAsChannelsFrameBased | Simulink:masks:ElementsAsChannelsSampleBased
      mask TypeOptions OutDataTypeStr: Simulink:masks:uint8 | Simulink:masks:boolean
      mask Display: fprintf('U > 0\n&  NOT\nU/z > 0')
  HDL Counter1 : hdlsllib/Sources/HDL Counter  CountType=Count limited  CountInit=1  CountStep=1  CountMax=2500000  CountFromType=Specify  CountFrom=1  CountResetPort=on  CountLoadPort=off  CountEnbPort=off  CountDirPort=off  CountHitOutputPort=off  CountDataType=Unsigned  CountWordLen=32  CountFracLen=0  CountSampTime=1
  Logical Operator3 : Logic  Operator=OR  AllPortsSameDT=off  OutDataTypeStr=boolean  SampleTime=1e-08
  Sum1 : Sum  OutDataTypeStr=uint32  AccumDataTypeStr=uint32  SampleTime=1e-08
  Switch10 : Switch  Criteria=u2 > Threshold  Threshold=double(0)  OutDataTypeStr=uint32  SampleTime=1e-08  SaturateOnIntegerOverflow=off  InputSameDT=off
  Switch11 : Switch  Criteria=u2 > Threshold  Threshold=double(0)  OutDataTypeStr=uint32  SampleTime=1e-08  SaturateOnIntegerOverflow=off  InputSameDT=off
  en_in_AXI_term1 : Terminator
  AXI_period : Outport  SampleTime=1e-08
  AXI_hightime : Outport  Port=2  SampleTime=1e-08
  AXI_lowtime : Outport  Port=3  SampleTime=1e-08
  wires:
  Switch10/1 -> Sum1/1, Delay12/1, Delay9/1
  Logical Operator3/1 -> HDL Counter1/1
  Delay15/1 -> Detect Rise Positive1/1(U), Detect Fall Nonpositive1/1(U)
  en_in_AXI/1 -> en_in_AXI_term1/1
  pwm_in/1 -> Delay15/1
  Detect Fall Nonpositive1/1(Y) -> Logical Operator3/2, Switch10/2
  Detect Rise Positive1/1(Y) -> Switch11/2, Logical Operator3/1
  HDL Counter1/1 -> Switch10/1, Switch11/1
  Switch11/1 -> Sum1/2, Delay11/1, Delay13/1
  Delay9/1 -> Switch10/3
  Delay12/1 -> AXI_hightime/1
  Sum1/1 -> Delay10/1
  Delay13/1 -> AXI_lowtime/1
  Delay11/1 -> Switch11/3
  Delay10/1 -> AXI_period/1

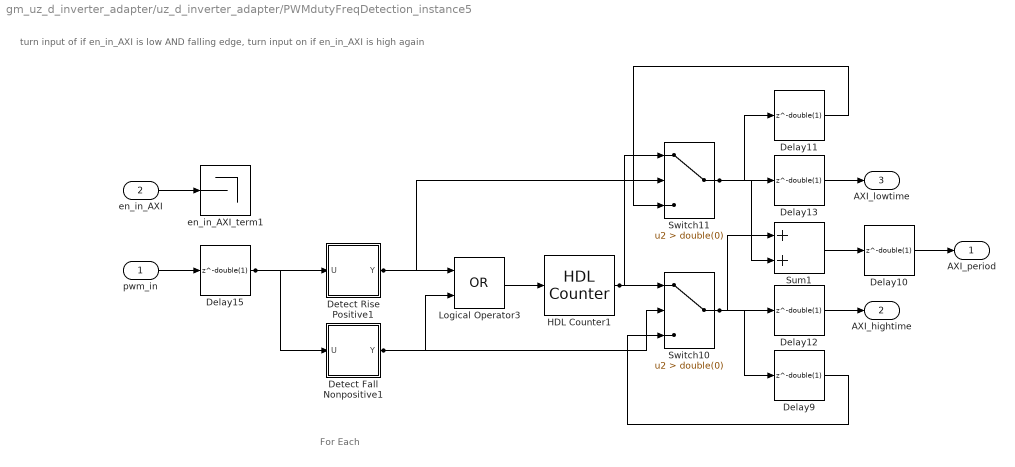
== system gm_uz_d_inverter_adapter/uz_d_inverter_adapter/PWMdutyFreqDetection_instance5 ==
  note: For Each
  note: turn input of if en_in_AXI is low AND falling edge, turn input on if en_in_AXI is high again
  pwm_in : Inport  OutDataTypeStr=fixdt(0, 1, 0)  PortDimensions=1  SampleTime=1e-08
  en_in_AXI : Inport  Port=2  OutDataTypeStr=boolean  PortDimensions=1  SampleTime=1e-08
  Delay{9..13,15} (6 alike) : Delay  DelayLength=double(1)  InitialCondition=0  SampleTime=1e-08
  Detect Fall Nonpositive1 : Subsystem  mask(Detect Fall Nonpositive){vinit=double(0), InputProcessing=Elements as channels (sample based), OutDataTypeStr=boolean}
      mask prompts: vinit "Simulink:masks:InitialCondition_MP"; InputProcessing "Simulink:masks:InputProcessing_MP"; OutDataTypeStr "Simulink:masks:OutputDataType_MP"
      mask help: Simulink:masks:DetectFallNonpositive_MD
      mask init:
      | InputProcessing = 'Elements as channels (sample based)';
      | OutDataTypeStr = 'boolean';
      | vinit = double(0);
      mask TypeOptions InputProcessing: Simulink:masks:ColumnsAsChannelsFrameBased | Simulink:masks:ElementsAsChannelsSampleBased
      mask TypeOptions OutDataTypeStr: Simulink:masks:uint8 | Simulink:masks:boolean
      mask Display: fprintf('U <= 0\n&  NOT\nU/z <= 0')
  Detect Rise Positive1 : Subsystem  mask(Detect Rise Positive){vinit=double(0), InputProcessing=Elements as channels (sample based), OutDataTypeStr=boolean}
      mask prompts: vinit "Simulink:masks:InitialCondition_MP"; InputProcessing "Simulink:masks:InputProcessing_MP"; OutDataTypeStr "Simulink:masks:OutputDataType_MP"
      mask help: Simulink:masks:DetectRisePositive_MD
      mask init:
      | InputProcessing = 'Elements as channels (sample based)';
      | OutDataTypeStr = 'boolean';
      | vinit = double(0);
      mask TypeOptions InputProcessing: Simulink:masks:ColumnsAsChannelsFrameBased | Simulink:masks:ElementsAsChannelsSampleBased
      mask TypeOptions OutDataTypeStr: Simulink:masks:uint8 | Simulink:masks:boolean
      mask Display: fprintf('U > 0\n&  NOT\nU/z > 0')
  HDL Counter1 : hdlsllib/Sources/HDL Counter  CountType=Count limited  CountInit=1  CountStep=1  CountMax=2500000  CountFromType=Specify  CountFrom=1  CountResetPort=on  CountLoadPort=off  CountEnbPort=off  CountDirPort=off  CountHitOutputPort=off  CountDataType=Unsigned  CountWordLen=32  CountFracLen=0  CountSampTime=1
  Logical Operator3 : Logic  Operator=OR  AllPortsSameDT=off  OutDataTypeStr=boolean  SampleTime=1e-08
  Sum1 : Sum  OutDataTypeStr=uint32  AccumDataTypeStr=uint32  SampleTime=1e-08
  Switch10 : Switch  Criteria=u2 > Threshold  Threshold=double(0)  OutDataTypeStr=uint32  SampleTime=1e-08  SaturateOnIntegerOverflow=off  InputSameDT=off
  Switch11 : Switch  Criteria=u2 > Threshold  Threshold=double(0)  OutDataTypeStr=uint32  SampleTime=1e-08  SaturateOnIntegerOverflow=off  InputSameDT=off
  en_in_AXI_term1 : Terminator
  AXI_period : Outport  SampleTime=1e-08
  AXI_hightime : Outport  Port=2  SampleTime=1e-08
  AXI_lowtime : Outport  Port=3  SampleTime=1e-08
  wires:
  en_in_AXI/1 -> en_in_AXI_term1/1
  Detect Fall Nonpositive1/1(Y) -> Switch10/2, Logical Operator3/2
  pwm_in/1 -> Delay15/1
  Logical Operator3/1 -> HDL Counter1/1
  Delay15/1 -> Detect Fall Nonpositive1/1(U), Detect Rise Positive1/1(U)
  Detect Rise Positive1/1(Y) -> Switch11/2, Logical Operator3/1
  HDL Counter1/1 -> Switch10/1, Switch11/1
  Switch11/1 -> Sum1/2, Delay13/1, Delay11/1
  Switch10/1 -> Sum1/1, Delay12/1, Delay9/1
  Delay11/1 -> Switch11/3
  Delay13/1 -> AXI_lowtime/1
  Delay10/1 -> AXI_period/1
  Sum1/1 -> Delay10/1
  Delay12/1 -> AXI_hightime/1
  Delay9/1 -> Switch10/3

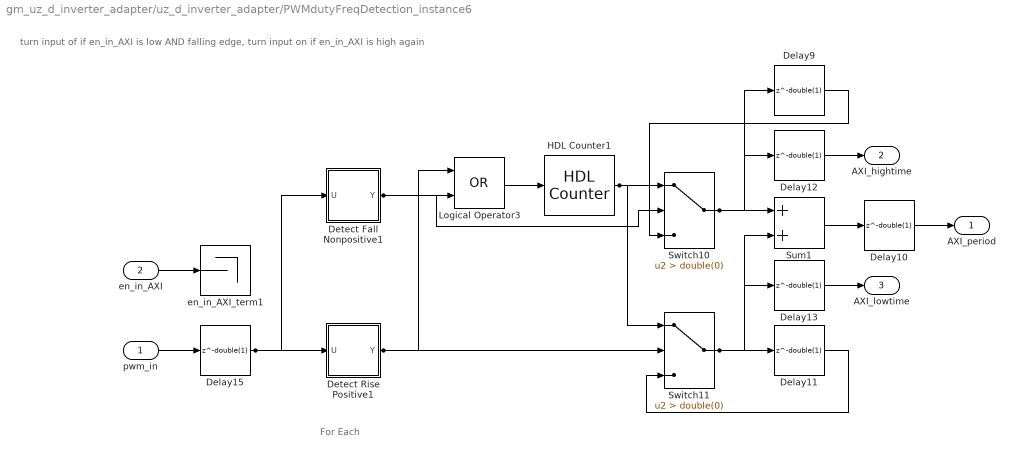
== system gm_uz_d_inverter_adapter/uz_d_inverter_adapter/PWMdutyFreqDetection_instance6 ==
  note: For Each
  note: turn input of if en_in_AXI is low AND falling edge, turn input on if en_in_AXI is high again
  pwm_in : Inport  OutDataTypeStr=fixdt(0, 1, 0)  PortDimensions=1  SampleTime=1e-08
  en_in_AXI : Inport  Port=2  OutDataTypeStr=boolean  PortDimensions=1  SampleTime=1e-08
  Delay{9..13,15} (6 alike) : Delay  DelayLength=double(1)  InitialCondition=0  SampleTime=1e-08
  Detect Fall Nonpositive1 : Subsystem  mask(Detect Fall Nonpositive){vinit=double(0), InputProcessing=Elements as channels (sample based), OutDataTypeStr=boolean}
      mask prompts: vinit "Simulink:masks:InitialCondition_MP"; InputProcessing "Simulink:masks:InputProcessing_MP"; OutDataTypeStr "Simulink:masks:OutputDataType_MP"
      mask help: Simulink:masks:DetectFallNonpositive_MD
      mask init:
      | InputProcessing = 'Elements as channels (sample based)';
      | OutDataTypeStr = 'boolean';
      | vinit = double(0);
      mask TypeOptions InputProcessing: Simulink:masks:ColumnsAsChannelsFrameBased | Simulink:masks:ElementsAsChannelsSampleBased
      mask TypeOptions OutDataTypeStr: Simulink:masks:uint8 | Simulink:masks:boolean
      mask Display: fprintf('U <= 0\n&  NOT\nU/z <= 0')
  Detect Rise Positive1 : Subsystem  mask(Detect Rise Positive){vinit=double(0), InputProcessing=Elements as channels (sample based), OutDataTypeStr=boolean}
      mask prompts: vinit "Simulink:masks:InitialCondition_MP"; InputProcessing "Simulink:masks:InputProcessing_MP"; OutDataTypeStr "Simulink:masks:OutputDataType_MP"
      mask help: Simulink:masks:DetectRisePositive_MD
      mask init:
      | InputProcessing = 'Elements as channels (sample based)';
      | OutDataTypeStr = 'boolean';
      | vinit = double(0);
      mask TypeOptions InputProcessing: Simulink:masks:ColumnsAsChannelsFrameBased | Simulink:masks:ElementsAsChannelsSampleBased
      mask TypeOptions OutDataTypeStr: Simulink:masks:uint8 | Simulink:masks:boolean
      mask Display: fprintf('U > 0\n&  NOT\nU/z > 0')
  HDL Counter1 : hdlsllib/Sources/HDL Counter  CountType=Count limited  CountInit=1  CountStep=1  CountMax=2500000  CountFromType=Specify  CountFrom=1  CountResetPort=on  CountLoadPort=off  CountEnbPort=off  CountDirPort=off  CountHitOutputPort=off  CountDataType=Unsigned  CountWordLen=32  CountFracLen=0  CountSampTime=1
  Logical Operator3 : Logic  Operator=OR  AllPortsSameDT=off  OutDataTypeStr=boolean  SampleTime=1e-08
  Sum1 : Sum  OutDataTypeStr=uint32  AccumDataTypeStr=uint32  SampleTime=1e-08
  Switch10 : Switch  Criteria=u2 > Threshold  Threshold=double(0)  OutDataTypeStr=uint32  SampleTime=1e-08  SaturateOnIntegerOverflow=off  InputSameDT=off
  Switch11 : Switch  Criteria=u2 > Threshold  Threshold=double(0)  OutDataTypeStr=uint32  SampleTime=1e-08  SaturateOnIntegerOverflow=off  InputSameDT=off
  en_in_AXI_term1 : Terminator
  AXI_period : Outport  SampleTime=1e-08
  AXI_hightime : Outport  Port=2  SampleTime=1e-08
  AXI_lowtime : Outport  Port=3  SampleTime=1e-08
  wires:
  en_in_AXI/1 -> en_in_AXI_term1/1
  Switch10/1 -> Delay12/1, Sum1/1, Delay9/1
  Detect Fall Nonpositive1/1(Y) -> Switch10/2, Logical Operator3/2
  pwm_in/1 -> Delay15/1
  Logical Operator3/1 -> HDL Counter1/1
  Delay15/1 -> Detect Fall Nonpositive1/1(U), Detect Rise Positive1/1(U)
  Detect Rise Positive1/1(Y) -> Switch11/2, Logical Operator3/1
  Delay11/1 -> Switch11/3
  HDL Counter1/1 -> Switch10/1, Switch11/1
  Switch11/1 -> Sum1/2, Delay11/1, Delay13/1
  Delay9/1 -> Switch10/3
  Delay12/1 -> AXI_hightime/1
  Sum1/1 -> Delay10/1
  Delay13/1 -> AXI_lowtime/1
  Delay10/1 -> AXI_period/1

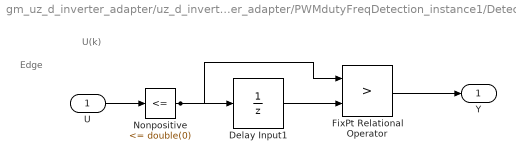
== system gm_uz_d_inverter_adapter/uz_d_inverter_adapter/PWMdutyFreqDetection_instance1/Detect Fall Nonpositive1 ==
  note: U(k)
  note: Edge
  U : Inport  OutDataTypeStr=fixdt(0, 1, 0)  SampleTime=1e-08
  Delay Input1 : UnitDelay  SampleTime=1e-08
  FixPt Relational Operator : RelationalOperator  Operator=>  OutDataTypeStr=boolean  SampleTime=1e-08  InputSameDT=off
  Nonpositive : simulink/Logic and Bit Operations/Compare To Constant  relop=<=  const=double(0)  OutDataTypeStr=boolean
  Y : Outport  SampleTime=1e-08
  wires:
  U/1 -> Nonpositive/1
  Nonpositive/1 -> FixPt Relational Operator/1, Delay Input1/1
  Delay Input1/1 -> FixPt Relational Operator/2
  FixPt Relational Operator/1 -> Y/1

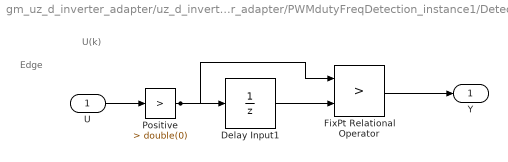
== system gm_uz_d_inverter_adapter/uz_d_inverter_adapter/PWMdutyFreqDetection_instance1/Detect Rise Positive1 ==
  note: U(k)
  note: Edge
  U : Inport  OutDataTypeStr=fixdt(0, 1, 0)  SampleTime=1e-08
  Delay Input1 : UnitDelay  SampleTime=1e-08
  FixPt Relational Operator : RelationalOperator  Operator=>  OutDataTypeStr=boolean  SampleTime=1e-08  InputSameDT=off
  Positive : simulink/Logic and Bit Operations/Compare To Constant  relop=>  const=double(0)  OutDataTypeStr=boolean
  Y : Outport  SampleTime=1e-08
  wires:
  U/1 -> Positive/1
  Positive/1 -> Delay Input1/1, FixPt Relational Operator/1
  Delay Input1/1 -> FixPt Relational Operator/2
  FixPt Relational Operator/1 -> Y/1

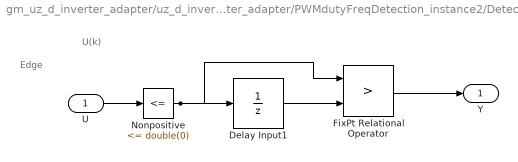
== system gm_uz_d_inverter_adapter/uz_d_inverter_adapter/PWMdutyFreqDetection_instance2/Detect Fall Nonpositive1 ==
  note: Edge
  note: U(k)
  U : Inport  OutDataTypeStr=fixdt(0, 1, 0)  SampleTime=1e-08
  Delay Input1 : UnitDelay  SampleTime=1e-08
  FixPt Relational Operator : RelationalOperator  Operator=>  OutDataTypeStr=boolean  SampleTime=1e-08  InputSameDT=off
  Nonpositive : simulink/Logic and Bit Operations/Compare To Constant  relop=<=  const=double(0)  OutDataTypeStr=boolean
  Y : Outport  SampleTime=1e-08
  wires:
  FixPt Relational Operator/1 -> Y/1
  Delay Input1/1 -> FixPt Relational Operator/2
  Nonpositive/1 -> Delay Input1/1, FixPt Relational Operator/1
  U/1 -> Nonpositive/1

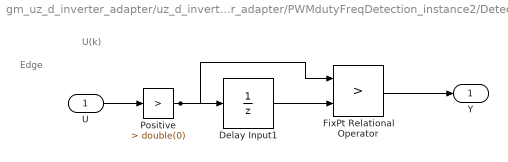
== system gm_uz_d_inverter_adapter/uz_d_inverter_adapter/PWMdutyFreqDetection_instance2/Detect Rise Positive1 ==
  note: Edge
  note: U(k)
  U : Inport  OutDataTypeStr=fixdt(0, 1, 0)  SampleTime=1e-08
  Delay Input1 : UnitDelay  SampleTime=1e-08
  FixPt Relational Operator : RelationalOperator  Operator=>  OutDataTypeStr=boolean  SampleTime=1e-08  InputSameDT=off
  Positive : simulink/Logic and Bit Operations/Compare To Constant  relop=>  const=double(0)  OutDataTypeStr=boolean
  Y : Outport  SampleTime=1e-08
  wires:
  FixPt Relational Operator/1 -> Y/1
  Delay Input1/1 -> FixPt Relational Operator/2
  Positive/1 -> FixPt Relational Operator/1, Delay Input1/1
  U/1 -> Positive/1

== system gm_uz_d_inverter_adapter/uz_d_inverter_adapter/PWMdutyFreqDetection_instance3/Detect Fall Nonpositive1 ==
  note: Edge
  note: U(k)
  U : Inport  OutDataTypeStr=fixdt(0, 1, 0)  SampleTime=1e-08
  Delay Input1 : UnitDelay  SampleTime=1e-08
  FixPt Relational Operator : RelationalOperator  Operator=>  OutDataTypeStr=boolean  SampleTime=1e-08  InputSameDT=off
  Nonpositive : simulink/Logic and Bit Operations/Compare To Constant  relop=<=  const=double(0)  OutDataTypeStr=boolean
  Y : Outport  SampleTime=1e-08
  wires:
  FixPt Relational Operator/1 -> Y/1
  Delay Input1/1 -> FixPt Relational Operator/2
  Nonpositive/1 -> Delay Input1/1, FixPt Relational Operator/1
  U/1 -> Nonpositive/1

== system gm_uz_d_inverter_adapter/uz_d_inverter_adapter/PWMdutyFreqDetection_instance3/Detect Rise Positive1 ==
  note: Edge
  note: U(k)
  U : Inport  OutDataTypeStr=fixdt(0, 1, 0)  SampleTime=1e-08
  Delay Input1 : UnitDelay  SampleTime=1e-08
  FixPt Relational Operator : RelationalOperator  Operator=>  OutDataTypeStr=boolean  SampleTime=1e-08  InputSameDT=off
  Positive : simulink/Logic and Bit Operations/Compare To Constant  relop=>  const=double(0)  OutDataTypeStr=boolean
  Y : Outport  SampleTime=1e-08
  wires:
  FixPt Relational Operator/1 -> Y/1
  Delay Input1/1 -> FixPt Relational Operator/2
  Positive/1 -> FixPt Relational Operator/1, Delay Input1/1
  U/1 -> Positive/1

== system gm_uz_d_inverter_adapter/uz_d_inverter_adapter/PWMdutyFreqDetection_instance4/Detect Fall Nonpositive1 ==
  note: Edge
  note: U(k)
  U : Inport  OutDataTypeStr=fixdt(0, 1, 0)  SampleTime=1e-08
  Delay Input1 : UnitDelay  SampleTime=1e-08
  FixPt Relational Operator : RelationalOperator  Operator=>  OutDataTypeStr=boolean  SampleTime=1e-08  InputSameDT=off
  Nonpositive : simulink/Logic and Bit Operations/Compare To Constant  relop=<=  const=double(0)  OutDataTypeStr=boolean
  Y : Outport  SampleTime=1e-08
  wires:
  FixPt Relational Operator/1 -> Y/1
  Delay Input1/1 -> FixPt Relational Operator/2
  Nonpositive/1 -> Delay Input1/1, FixPt Relational Operator/1
  U/1 -> Nonpositive/1

== system gm_uz_d_inverter_adapter/uz_d_inverter_adapter/PWMdutyFreqDetection_instance4/Detect Rise Positive1 ==
  note: Edge
  note: U(k)
  U : Inport  OutDataTypeStr=fixdt(0, 1, 0)  SampleTime=1e-08
  Delay Input1 : UnitDelay  SampleTime=1e-08
  FixPt Relational Operator : RelationalOperator  Operator=>  OutDataTypeStr=boolean  SampleTime=1e-08  InputSameDT=off
  Positive : simulink/Logic and Bit Operations/Compare To Constant  relop=>  const=double(0)  OutDataTypeStr=boolean
  Y : Outport  SampleTime=1e-08
  wires:
  FixPt Relational Operator/1 -> Y/1
  Delay Input1/1 -> FixPt Relational Operator/2
  Positive/1 -> FixPt Relational Operator/1, Delay Input1/1
  U/1 -> Positive/1

== system gm_uz_d_inverter_adapter/uz_d_inverter_adapter/PWMdutyFreqDetection_instance5/Detect Fall Nonpositive1 ==
  note: Edge
  note: U(k)
  U : Inport  OutDataTypeStr=fixdt(0, 1, 0)  SampleTime=1e-08
  Delay Input1 : UnitDelay  SampleTime=1e-08
  FixPt Relational Operator : RelationalOperator  Operator=>  OutDataTypeStr=boolean  SampleTime=1e-08  InputSameDT=off
  Nonpositive : simulink/Logic and Bit Operations/Compare To Constant  relop=<=  const=double(0)  OutDataTypeStr=boolean
  Y : Outport  SampleTime=1e-08
  wires:
  FixPt Relational Operator/1 -> Y/1
  Delay Input1/1 -> FixPt Relational Operator/2
  Nonpositive/1 -> Delay Input1/1, FixPt Relational Operator/1
  U/1 -> Nonpositive/1

== system gm_uz_d_inverter_adapter/uz_d_inverter_adapter/PWMdutyFreqDetection_instance5/Detect Rise Positive1 ==
  note: Edge
  note: U(k)
  U : Inport  OutDataTypeStr=fixdt(0, 1, 0)  SampleTime=1e-08
  Delay Input1 : UnitDelay  SampleTime=1e-08
  FixPt Relational Operator : RelationalOperator  Operator=>  OutDataTypeStr=boolean  SampleTime=1e-08  InputSameDT=off
  Positive : simulink/Logic and Bit Operations/Compare To Constant  relop=>  const=double(0)  OutDataTypeStr=boolean
  Y : Outport  SampleTime=1e-08
  wires:
  FixPt Relational Operator/1 -> Y/1
  Delay Input1/1 -> FixPt Relational Operator/2
  Positive/1 -> FixPt Relational Operator/1, Delay Input1/1
  U/1 -> Positive/1

== system gm_uz_d_inverter_adapter/uz_d_inverter_adapter/PWMdutyFreqDetection_instance6/Detect Fall Nonpositive1 ==
  note: Edge
  note: U(k)
  U : Inport  OutDataTypeStr=fixdt(0, 1, 0)  SampleTime=1e-08
  Delay Input1 : UnitDelay  SampleTime=1e-08
  FixPt Relational Operator : RelationalOperator  Operator=>  OutDataTypeStr=boolean  SampleTime=1e-08  InputSameDT=off
  Nonpositive : simulink/Logic and Bit Operations/Compare To Constant  relop=<=  const=double(0)  OutDataTypeStr=boolean
  Y : Outport  SampleTime=1e-08
  wires:
  FixPt Relational Operator/1 -> Y/1
  Delay Input1/1 -> FixPt Relational Operator/2
  Nonpositive/1 -> Delay Input1/1, FixPt Relational Operator/1
  U/1 -> Nonpositive/1

== system gm_uz_d_inverter_adapter/uz_d_inverter_adapter/PWMdutyFreqDetection_instance6/Detect Rise Positive1 ==
  note: Edge
  note: U(k)
  U : Inport  OutDataTypeStr=fixdt(0, 1, 0)  SampleTime=1e-08
  Delay Input1 : UnitDelay  SampleTime=1e-08
  FixPt Relational Operator : RelationalOperator  Operator=>  OutDataTypeStr=boolean  SampleTime=1e-08  InputSameDT=off
  Positive : simulink/Logic and Bit Operations/Compare To Constant  relop=>  const=double(0)  OutDataTypeStr=boolean
  Y : Outport  SampleTime=1e-08
  wires:
  FixPt Relational Operator/1 -> Y/1
  Delay Input1/1 -> FixPt Relational Operator/2
  Positive/1 -> FixPt Relational Operator/1, Delay Input1/1
  U/1 -> Positive/1
